simulink model "FarrowResamp"  (Simulink 6.6)
settings: Solver=VariableStepDiscrete  StartTime=0.0  StopTime=1800*clock_sample  RelTol=1e-3
PreLoadFcn:
  | clock_period=50/3
  | clock_sample=clock_period*1.0e-009
  | slow_clock=25
  | fast_clock=32
InitFcn:
  | %% DSPBuilder Start
  | alt_dspbuilder_update_model(bdroot)
  | %% DSPBuilder End
undefined symbols (not defined in the file): get
libraries: allblocks_alteradspbuilder2 x65, dspsnks4 x4
settings Model: Creator=mjervis  LastModifiedBy=lkong
settings DataIOCC: SignalLoggingName=sigsOut
settings OptimizationCC: InlineInvariantSignals=on
settings DebuggingCC: SignalResolutionControl=TryResolveAllWithWarning  SolverPrmCheckMsg=none  MultiTaskDSMMsg=warning  MultiTaskCondExecSysMsg=none  SigSpecEnsureSampleTimeMsg=none
settings HardwareCC: TargetUnknown=on
settings RTWCC: IncludeERTFirstTime=on

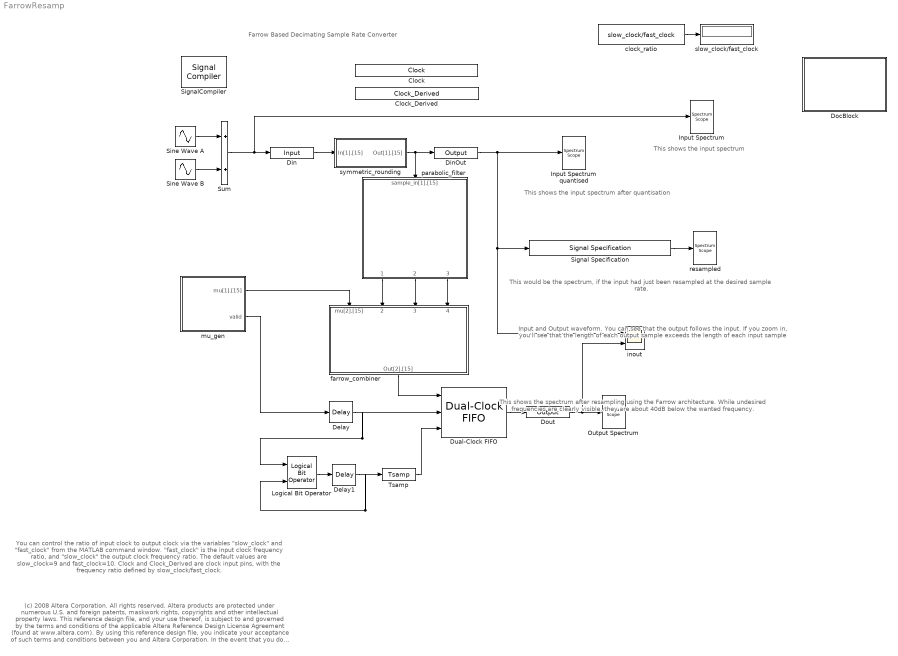
== system FarrowResamp ==
  note: (c) 2008 Altera Corporation. All rights reserved.  Altera products are protected under numerous U.S. and foreign patents, maskwork rights, copyrights and other intellectual property laws.
      | This reference design file, and your use thereof, is subject to and governed by the terms and conditions of the applicable Altera Reference Design License Agreement (found at www.altera.com).
      | By using this reference design file, you indicate your acceptance of such terms and conditions between you and Altera Corporation.
      | In the event that you do not agree with such terms and conditions, you may not use the reference design file and please promptly destroy any copies you have made.
      | This reference design file being provided on an "as-is" basis and as an accommodation and therefore all warranties, representations or guarantees of any kind (whether express, implied or statutory)
      | including, without limitation, warranties of merchantability, non-infringement, or fitness for a particular purpose, are specifically disclaimed.
      | By making this reference design file available, Altera expressly does not recommend, suggest or require that this reference design file be used in combination with any other product not provided by Altera
  note: This shows the input spectrum
  note: This shows the input spectrum after quantisation
  note: This shows the spectrum after resampling using the Farrow
      | architecture.  While undesired frequencies are clearly visible,
      | they are about 40dB below the wanted frequency.
  note: You can control the ratio of input clock to output clock via the variables "slow_clock" and "fast_clock" from the
      | MATLAB command window.  "fast_clock" is the input clock frequency ratio, and "slow_clock" the output clock
      | frequency ratio. The default values are slow_clock=9 and fast_clock=10.
      |
      | Clock and Clock_Derived are clock input pins, with the frequency ratio defined by slow_clock/fast_clock.
  note: Farrow Based Decimating Sample Rate Converter
  note: This would be the spectrum, if the input had
      | just been resampled at the desired sample rate.
  note: Input and Output waveform.  You can see that the output
      | follows the input.  If you zoom in, you'll see that the length
      | of each output sample exceeds the length of each input
      | sample
  Clock : allblocks_alteradspbuilder2/Clock  ClockPeriod=clock_period  ClockPeriodUnit=ns  SampleTime=clock_sample  SimulationStartCycle=5  PhaseOffset=0  Reset=aclr  ResetType=Active Low  Export=off
  Clock_Derived : allblocks_alteradspbuilder2/Clock_Derived  ClockNumerator=slow_clock  ClockDenominator=fast_clock  SimulationStartCycle=5  PhaseOffset=0  Reset=slow_aclr  ResetType=Active Low  Export=off
  Delay : allblocks_alteradspbuilder2/Delay  pipeline=4  pipeline_display=4  ClockPhase=1  use_ena=off  use_sclr=off  allowFloatingPointOverride=on  logOutputs=off  logFile=d:\spr\269066\tb_FarrowResamp\FarrowResamp_Delay.fixedpointlog  use_init=off  reset_value=1
  Delay1 : allblocks_alteradspbuilder2/Delay  pipeline=4  pipeline_display=4  ClockPhase=1  use_ena=off  use_sclr=off  allowFloatingPointOverride=on  logOutputs=off  logFile=d:\spr\269066\tb_FarrowResamp\FarrowResamp_Delay1.fixedpointlog  use_init=off  reset_value=1
  Din : allblocks_alteradspbuilder2/Input  iofile=d:\spr\269066\tb_FarrowResamp\FarrowResamp_Din.salt  BusType=Signed Fractional  bwl=1  bwr=15  SpecifyClock=on  clock=Clock  PORTTYPE=Input  externalType=Inferred  allowFloatingPointOverride=on  logOutputs=off
  DinOut : allblocks_alteradspbuilder2/Output  iofile=d:\spr\269066\tb_FarrowResamp\FarrowResamp_DinOut.capture  BusType=Signed Fractional  bwl=1  bwr=15  externalType=Inferred  PORTTYPE=Output  allowFloatingPointOverride=on  logOutputs=off
  DocBlock : Subsystem  mask(DocBlock){ECoderFlag=, DocumentType=Text}
      content=|
      | =============================================
      | Farrow Based Decimating Sample Rate Converter
      | =============================================
      |
      | Introduction
      | ------------
      | Many integrated systems, such as Software Defined Radios (SDR), require data
      | to be resampled.  This is typically the case where a unit can be configured to
      | comply with different communication standards, where the sample rates are different.
      | In some cases, where one clock rate is a simple integer multiply of another clock
      | rate, this can be done with interpolating and decimating FIR filters.  However, in
      | most cases the interpolation and decimation factors would be so high that this
      | approach is impractical.
      | Farrow resamplers offer an efficient way to resample a data stream at a different
      | sample rate.  The underlying principle is that the phase difference between the
      | current input and wanted output is determined on a sample by sample basis.  This
      | phase difference is then used to combine the phases of a polyphase filter in such
      | a way that a sample for the wanted output phase is generated.
      | This design demonstrates how a Farrow resampler is working.  You can simulate its
      | performance in MATLAB, change it as required for your application, generate a
      | VDHL version and synthesize it to Altera devices.
      | This demo is designed for an input clock rate identical to the system clock.  For
      | applications where the input rate is much lower than the system clock, time sharing
      | should be implemented to get a cost effective solution.
      |
      |
      | Usage
      | -----
      | You can run the design as it is, just press the run button to start the simulation.
      | You will get 4 waveforms, showing the spectrum at the following places:
      | 1) the input
      | 2) the input, quantised
      | 3) the input, if it had been just resampledby registering it in a flip flop running
      |    at the output clock rate (the simplest way of changing sample rate)
      | 4) at the output of the Farrow resampler.
      |
      | You can generate VHDL and synthesise the same way as any other DSPBuilder design
      | using the "SignalCompiler" block.
      |
      | You can change the stimuli by connecting the input to a different source.  If you
      | want to change the ratio of input clock to output clock, you can do this from the
      | MATLAB command prompt.  In this case, please set the variables "slow_clock" and
      | "fast_clock" to the required numbers, by default they are set to 9 and 10 to provide
      | a ratio of 9/10, i.e. the output rate is 90% of the input clock rate.  The
      | variables "fast_clock" and "slow_clock" are used in a number of instances
      | throughout the design.  The rules for setting these variables are:
      | 1) slow_clock, i.e. the output clock, must be slower than fast_clock for a deci-
      |    mating Farrow filter.
      | 2) slow_clock*fast_clock must be less than 2^14.  This is a restriction of this
      |    particular implementation.  You can work with ratios where this is not the
      |    case, but you then need to change the bit width in the accumulators in the
      |    mu_gen block.
      | 3) If slow_clock is less than half of fast_clock, the filter will work, but
      |    the results will be sub-optimal.  In this case it is better to double slow_clock,
      |    which should then still be less than fast_clock, and decimate at the output by
      |    rejecting every other sample.
      |
      |
      | Design details
      | --------------
      |
      | Input Stimuli
      |
      |   This testbench provides three stimuli:
      |   1) The sinewave generator is useful to analyse the effect of the resampling on
      |      the frequency spectrum.   You can change the frequency by double-clicking
      |      the "Sine Wave" block, and changing the "Samples per Period" parameter.
      |   2) The impulse generator generates a single impulse and is 0 for the rest of the
      |      simulation.  This is a useful tool for investigating the filter, which is part
      |      of the farrow resampler.
      |   3) The addition of two sinewaves.
      |
      | Symmetric rounding
      |
      |   Symmetric rounding ensures that no DC offset is introduced through the
      |   rounding operation.
      |
      | Parabolic filter
      |
      |   Low pass filter with passband=0.25 and stopband=0.75 .  You find more detailed
      |   documentation when you push into the filter by double-clicking it.
      |
      | mu Generator
      |
      |   This block calculates the phase difference between the current input sample
      |   and the desired output sample.  Double-click for more information.
      |
      | Farrow Combiner
      |
      |   The farrow combiner replaces the polyphase selector in traditional polyphase
      |   filters.  It will weigh the individual polyphases before adding them.  Double-
      |   click the Farrow_Combiner block for more information.
      |
      | FIFO
      |
      |   The farrow combiner works at the input clock rate.  This means it generates more
      |   samples than it should.  The task of the FIFO is to remove invalid samples, and
      |   also allows the transfer between the clock domains.  While the write side works
      |   at input clock rate, the read side works at output clock rate.
      mask prompts: ECoderFlag "E Coder Flag"; DocumentType "Document Type"
      mask help: Use this block to save long descriptive text with the model. Double-clicking the block will open an editor.
      settings: CopyFcn=docblock('breaklink',gcb);  DeleteFcn=docblock('close_document',gcb);  PreSaveFcn=docblock('save_document',gcb);  OpenFcn=docblock('edit_document',gcb);
      mask StyleString: edit,popup(Text|RTF|HTML)
      mask Display:
      | plot([.8 0 0 1 1 .8 .8 1],[1 1 0 0 .8 1 .8 .8]);
      | text(.5,.5,'DOC','horizontalalignment','center');
  Dout : allblocks_alteradspbuilder2/Output  iofile=d:\spr\269066\tb_FarrowResamp\FarrowResamp_Dout.capture  BusType=Signed Fractional  bwl=2  bwr=15  externalType=Inferred  PORTTYPE=Output  allowFloatingPointOverride=on  logOutputs=off
  Dual-Clock FIFO : allblocks_alteradspbuilder2/Dual-Clock FIFO  numwords=16  BusType=Signed Fractional  bwl=2  bwr=15  ram_type=AUTO  UseBaseWriteClock=on  UseBaseReadClock=off  read_clock=Clock_Derived  use_rdempty=off  use_rdfull=off  use_rdusedw=off  use_wrempty=off  use_wrfull=off  use_wrusedw=off  use_user_aclr=off  register_output=off  use_les_only=off  showahead_mode=off  synchronized=off  allowFloatingPointOverride=on  logOutputs=off  logFile=d:\spr\269066\tb_FarrowResamp\FarrowResamp_Dual-Clock+FIFO.fixedpointlog
  Input Spectrum : dspsnks4/Spectrum Scope  DialogController=dspdialog.SpectrumScope  DialogControllerArgs=DataTag1  SystemSampleTime=-1  ScopeProperties=on  Domain=Frequency  HorizSpan=1  UseBuffer=on  BufferSize=1024  Overlap=512  inpFftLenInherit=off  FFTlength=128  numAvg=2  DisplayProperties=off  AxisGrid=on  Memory=off  FrameNumber=on  AxisLegend=off  AxisZoom=off  OpenScopeAtSimStart=on  OpenScopeImmediately=off  FigPos=get(0,'defaultfigureposition')  AxisProperties=off  XUnits=Hertz  XRange=[0...Fs/2]  InheritXIncr=on  XIncr=1.0  XLabel=Samples  XLimit=Auto  YUnits=dB  XMax=1  XMin=0  YLabel=Magnitude, dB  LineProperties=off  wintypeSpecScope=Hann  RsSpecScope=50  betaSpecScope=5  winsampSpecScope=Periodic
      settings: YMin=-153.243329043552  YMax=22.477497462716
  Input Spectrum quantised : dspsnks4/Spectrum Scope  DialogController=dspdialog.SpectrumScope  DialogControllerArgs=DataTag2  SystemSampleTime=-1  ScopeProperties=on  Domain=Frequency  HorizSpan=1  UseBuffer=on  BufferSize=1024  Overlap=512  inpFftLenInherit=off  FFTlength=128  numAvg=2  DisplayProperties=off  AxisGrid=on  Memory=off  FrameNumber=on  AxisLegend=off  AxisZoom=off  OpenScopeAtSimStart=on  OpenScopeImmediately=off  FigPos=get(0,'defaultfigureposition')  AxisProperties=off  XUnits=Hertz  XRange=[0...Fs/2]  InheritXIncr=on  XIncr=1.0  XLabel=Samples  XLimit=Auto  YUnits=dB  XMax=1  XMin=0  YLabel=Magnitude, dB  LineProperties=off  LineColors=magenta  wintypeSpecScope=Hann  RsSpecScope=50  betaSpecScope=5  winsampSpecScope=Periodic
      settings: YMin=-152.110626534928  YMax=22.4774480317679
  Logical Bit Operator : allblocks_alteradspbuilder2/Logical Bit Operator  LogicalOperator=OR  user_inputs=2  pipeline_display=0
  Output Spectrum : dspsnks4/Spectrum Scope  DialogController=dspdialog.SpectrumScope  DialogControllerArgs=DataTag3  SystemSampleTime=-1  ScopeProperties=on  Domain=Frequency  HorizSpan=1  UseBuffer=on  BufferSize=1024  Overlap=512  inpFftLenInherit=off  FFTlength=128  numAvg=2  DisplayProperties=off  AxisGrid=on  Memory=off  FrameNumber=on  AxisLegend=off  AxisZoom=off  OpenScopeAtSimStart=on  OpenScopeImmediately=off  FigPos=get(0,'defaultfigureposition')  AxisProperties=off  XUnits=Hertz  XRange=[0...Fs/2]  InheritXIncr=on  XIncr=1.0  XLabel=Samples  XLimit=Auto  YUnits=dB  XMax=1  XMin=0  YLabel=Magnitude, dB  LineProperties=off  LineColors=blue  wintypeSpecScope=Hann  RsSpecScope=50  betaSpecScope=5  winsampSpecScope=Periodic
      settings: YMin=-107.092610263266  YMax=23.1676114232961
  Signal Specification : SignalSpecification  SampleTime=clock_sample * (slow_clock/fast_clock)
  SignalCompiler : allblocks_alteradspbuilder2/Signal Compiler  DeviceFamily=Stratix III  DeviceName=AUTO  EnableSignalTap=off  SignalTapDepth=128  UseBoardBlock=off  StpUseDefaultClock=on  StpClock=clock  ExportDir=.
  Sine Wave A : Sin  SineType=Sample based  Amplitude=0.4999  SampleTime=clock_sample
  Sine Wave B : Sin  SineType=Sample based  Amplitude=0.4999  Samples=11  SampleTime=clock_sample
  Sum : Sum  SaturateOnIntegerOverflow=on
  Tsamp : allblocks_alteradspbuilder2/Tsamp  SpecifyClock=on  clock=Clock_Derived
  clock_ratio : Constant  Value=slow_clock/fast_clock
  farrow_combiner : Subsystem  Orientation=down  AncestorBlock=ALTELINK/AltLab/HDL SubSystem
      mask Type: SubSystem AlteraBlockSet
  inout : Scope  NumInputPorts=2
      settings: YMin=-5~-5  YMax=5~5  SaveName=ScopeData2
  mu_gen : Subsystem  AncestorBlock=ALTELINK/AltLab/HDL SubSystem
      mask Type: SubSystem AlteraBlockSet
  parabolic_filter : Subsystem  Orientation=down  AncestorBlock=ALTELINK/AltLab/HDL SubSystem
      mask Type: SubSystem AlteraBlockSet
  resampled : dspsnks4/Spectrum Scope  DialogController=dspdialog.SpectrumScope  DialogControllerArgs=DataTag4  SystemSampleTime=-1  ScopeProperties=on  Domain=Frequency  HorizSpan=1  UseBuffer=on  BufferSize=1024  Overlap=512  inpFftLenInherit=off  FFTlength=128  numAvg=2  DisplayProperties=off  AxisGrid=on  Memory=off  FrameNumber=on  AxisLegend=off  AxisZoom=off  OpenScopeAtSimStart=on  OpenScopeImmediately=off  FigPos=get(0,'defaultfigureposition')  AxisProperties=off  XUnits=Hertz  XRange=[0...Fs/2]  InheritXIncr=on  XIncr=1.0  XLabel=Samples  XLimit=Auto  YUnits=dB  XMax=1  XMin=0  YLabel=Magnitude, dB  LineProperties=off  LineColors=magenta  wintypeSpecScope=Hann  RsSpecScope=50  betaSpecScope=5  winsampSpecScope=Periodic
      settings: YMin=-152.110626534928  YMax=22.4774480317679
  slow_clock/fast_clock : Display
  symmetric_rounding : Subsystem  AncestorBlock=ALTELINK/AltLab/HDL SubSystem
      mask Type: SubSystem AlteraBlockSet
  wires:
  parabolic_filter/1(phase0[3].[15]) -> farrow_combiner/2(phase0[3].[15])
  parabolic_filter/2(phase1[3].[15]) -> farrow_combiner/3(phase1[3].[15])
  parabolic_filter/3(phase2[3].[15]) -> farrow_combiner/4(phase2[2].[15])
  mu_gen/1(mu[1].[15]) -> farrow_combiner/1(mu[2].[15])
  mu_gen/2(valid) -> Delay/1
  Delay/1 -> Dual-Clock FIFO/2, Logical Bit Operator/1
  Dout/1 -> Output Spectrum/1, inout/2
  Din/1 -> symmetric_rounding/1(In[1].[15])
  clock_ratio/1 -> slow_clock/fast_clock/1
  Sine Wave A/1 -> Sum/1
  Sine Wave B/1 -> Sum/2
  Signal Specification/1 -> resampled/1
  symmetric_rounding/1(Out[1].[15]) -> parabolic_filter/1(sample_in[1].[15]), DinOut/1
  Sum/1 -> Din/1, Input Spectrum/1
  DinOut/1 -> Input Spectrum quantised/1, inout/1, Signal Specification/1
  Logical Bit Operator/1 -> Delay1/1
  Delay1/1 -> Logical Bit Operator/2, Tsamp/1
  Tsamp/1 -> Dual-Clock FIFO/3
  Dual-Clock FIFO/1 -> Dout/1
  farrow_combiner/1(Out[2].[15]) -> Dual-Clock FIFO/1

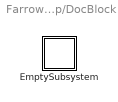
== system FarrowResamp/DocBlock ==
  EmptySubsystem : Subsystem

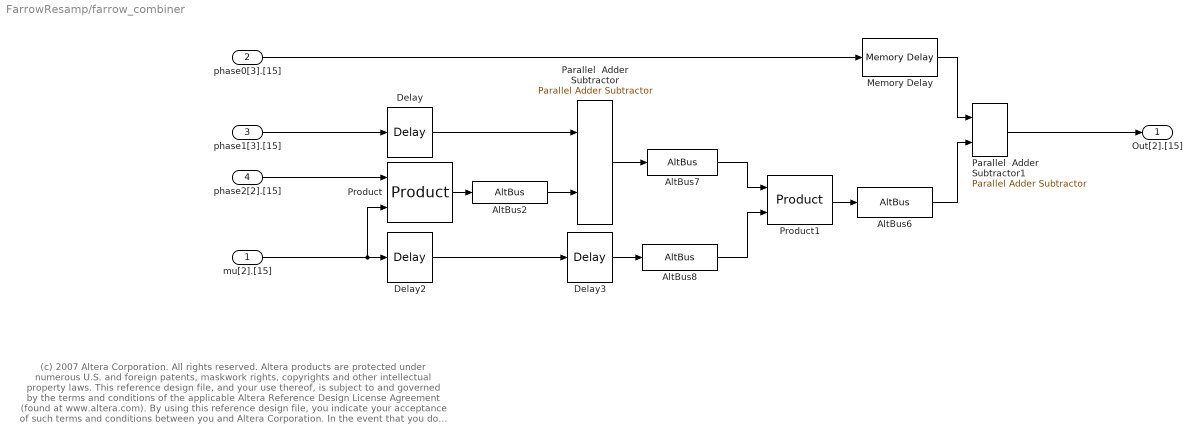
== system FarrowResamp/farrow_combiner ==
  note: (c) 2007 Altera Corporation. All rights reserved.  Altera products are protected under numerous U.S. and foreign patents, maskwork rights, copyrights and other intellectual property laws.
      | This reference design file, and your use thereof, is subject to and governed by the terms and conditions of the applicable Altera Reference Design License Agreement (found at www.altera.com).
      | By using this reference design file, you indicate your acceptance of such terms and conditions between you and Altera Corporation.
      | In the event that you do not agree with such terms and conditions, you may not use the reference design file and please promptly destroy any copies you have made.
      | This reference design file being provided on an "as-is" basis and as an accommodation and therefore all warranties, representations or guarantees of any kind (whether express, implied or statutory)
      | including, without limitation, warranties of merchantability, non-infringement, or fitness for a particular purpose, are specifically disclaimed.
      | By making this reference design file available, Altera expressly does not recommend, suggest or require that this reference design file be used in combination with any other product not provided by Altera
  mu[2].[15] : Inport
  phase0[3].[15] : Inport  Port=2
  phase1[3].[15] : Inport  Port=3
  phase2[2].[15] : Inport  Port=4
  AltBus2 : allblocks_alteradspbuilder2/AltBus  BusType=Signed Fractional  bwl=3  bwr=15  saturate=off  floatingPointInput=off  floatingPointOutput=off  logOutputs=off  logFile=d:\spr\269066\tb_FarrowResamp\FarrowResamp_farrow%5Fcombiner_AltBus2.fixedpointlog
  AltBus6 : allblocks_alteradspbuilder2/AltBus  BusType=Signed Fractional  bwl=5  bwr=15  saturate=off  floatingPointInput=off  floatingPointOutput=off  logOutputs=off  logFile=d:\spr\269066\tb_FarrowResamp\FarrowResamp_farrow%5Fcombiner_AltBus6.fixedpointlog
  AltBus7 : allblocks_alteradspbuilder2/AltBus  BusType=Signed Fractional  bwl=3  bwr=15  saturate=on  floatingPointInput=off  floatingPointOutput=off  logOutputs=off  logFile=d:\spr\269066\tb_FarrowResamp\FarrowResamp_farrow%5Fcombiner_AltBus7.fixedpointlog
  AltBus8 : allblocks_alteradspbuilder2/AltBus  BusType=Signed Fractional  bwl=2  bwr=15  saturate=off  floatingPointInput=off  floatingPointOutput=off  logOutputs=off  logFile=d:\spr\269066\tb_FarrowResamp\FarrowResamp_farrow%5Fcombiner_AltBus8.fixedpointlog
  Delay : allblocks_alteradspbuilder2/Delay  pipeline=1  pipeline_display=1  ClockPhase=1  use_ena=off  use_sclr=off  allowFloatingPointOverride=on  logOutputs=off  logFile=d:\spr\269066\tb_FarrowResamp\FarrowResamp_farrow%5Fcombiner_Delay.fixedpointlog  use_init=off  reset_value=1
  Delay2 : allblocks_alteradspbuilder2/Delay  pipeline=1  pipeline_display=1  ClockPhase=1  use_ena=off  use_sclr=off  allowFloatingPointOverride=on  logOutputs=off  logFile=d:\spr\269066\tb_FarrowResamp\FarrowResamp_farrow%5Fcombiner_Delay2.fixedpointlog  use_init=off  reset_value=1
  Delay3 : allblocks_alteradspbuilder2/Delay  pipeline=1  pipeline_display=1  ClockPhase=1  use_ena=off  use_sclr=off  allowFloatingPointOverride=on  logOutputs=off  logFile=d:\spr\269066\tb_FarrowResamp\FarrowResamp_farrow%5Fcombiner_Delay3.fixedpointlog  use_init=off  reset_value=1
  Memory Delay : allblocks_alteradspbuilder2/Memory Delay  BusType=Inferred  bwl=8  bwr=0  pipeline=3  pipeline_display=3  ram_type=AUTO  use_ena=off  use_sclr=off  allowFloatingPointOverride=on  logOutputs=off  logFile=d:\spr\269066\tb_FarrowResamp\FarrowResamp_farrow%5Fcombiner_Memory+Delay.fixedpointlog
  Parallel  Adder Subtractor : allblocks_alteradspbuilder2/Parallel Adder Subtractor  number_of_inputs=2  direction=++  use_pipeline=on  pipeline_display=1  phase_selection=1  use_ena=off  use_aclr=off  allowFloatingPointOverride=on  logOutputs=off  logFile=d:\spr\269066\tb_FarrowResamp\FarrowResamp_farrow%5Fcombiner_Parallel+%0AAdder+Subtractor.fixedpointlog
  Parallel  Adder Subtractor1 : allblocks_alteradspbuilder2/Parallel Adder Subtractor  number_of_inputs=2  direction=++  use_pipeline=on  pipeline_display=1  phase_selection=1  use_ena=off  use_aclr=off  allowFloatingPointOverride=on  logOutputs=off  logFile=d:\spr\269066\tb_FarrowResamp\FarrowResamp_farrow%5Fcombiner_Parallel+%0AAdder+Subtractor1.fixedpointlog
  Product : allblocks_alteradspbuilder2/Product  BusType=Inferred  bwl=8  bwr=0  pipeline=1  pipeline_display=1  phase_selection=1  use_ena=off  use_aclr=off  UseLPM=off  UseDedicatedCircuitry=off  allowFloatingPointOverride=on  logOutputs=off  logFile=d:\spr\269066\tb_FarrowResamp\FarrowResamp_farrow%5Fcombiner_Product.fixedpointlog
  Product1 : allblocks_alteradspbuilder2/Product  BusType=Inferred  bwl=8  bwr=0  pipeline=1  pipeline_display=1  phase_selection=1  use_ena=off  use_aclr=off  UseLPM=off  UseDedicatedCircuitry=off  allowFloatingPointOverride=on  logOutputs=off  logFile=d:\spr\269066\tb_FarrowResamp\FarrowResamp_farrow%5Fcombiner_Product1.fixedpointlog
  Out[2].[15] : Outport
  wires:
  phase0[3].[15]/1 -> Memory Delay/1
  phase1[3].[15]/1 -> Delay/1
  phase2[2].[15]/1 -> Product/1
  mu[2].[15]/1 -> Product/2, Delay2/1
  Delay/1 -> Parallel  Adder Subtractor/1
  Product/1 -> AltBus2/1
  Parallel  Adder Subtractor/1 -> AltBus7/1
  Delay2/1 -> Delay3/1
  Product1/1 -> AltBus6/1
  Delay3/1 -> AltBus8/1
  AltBus8/1 -> Product1/2
  AltBus6/1 -> Parallel  Adder Subtractor1/2
  AltBus7/1 -> Product1/1
  Parallel  Adder Subtractor1/1 -> Out[2].[15]/1
  Memory Delay/1 -> Parallel  Adder Subtractor1/1
  AltBus2/1 -> Parallel  Adder Subtractor/2

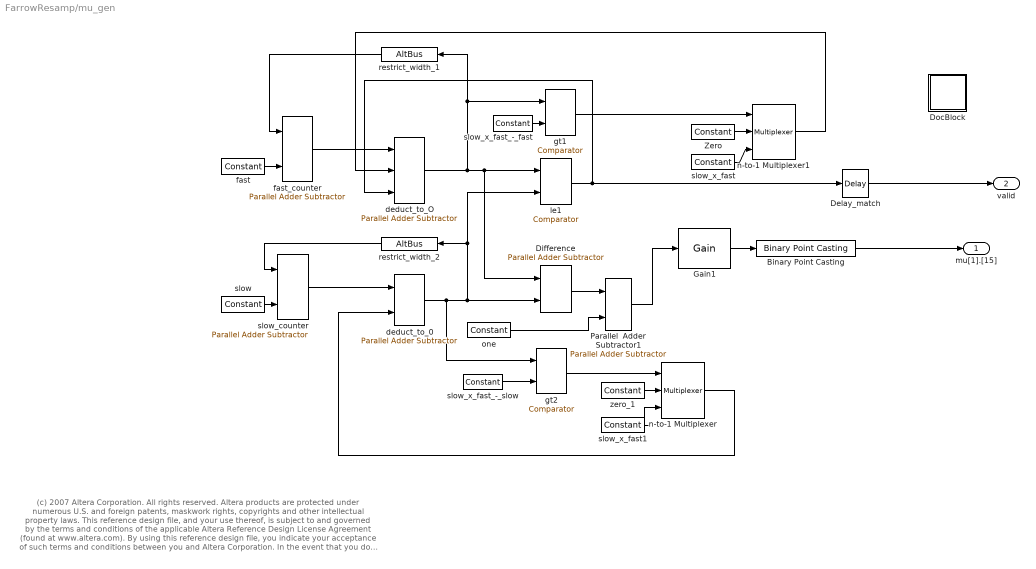
== system FarrowResamp/mu_gen ==
  note: (c) 2007 Altera Corporation. All rights reserved.  Altera products are protected under numerous U.S. and foreign patents, maskwork rights, copyrights and other intellectual property laws.
      | This reference design file, and your use thereof, is subject to and governed by the terms and conditions of the applicable Altera Reference Design License Agreement (found at www.altera.com).
      | By using this reference design file, you indicate your acceptance of such terms and conditions between you and Altera Corporation.
      | In the event that you do not agree with such terms and conditions, you may not use the reference design file and please promptly destroy any copies you have made.
      | This reference design file being provided on an "as-is" basis and as an accommodation and therefore all warranties, representations or guarantees of any kind (whether express, implied or statutory)
      | including, without limitation, warranties of merchantability, non-infringement, or fitness for a particular purpose, are specifically disclaimed.
      | By making this reference design file available, Altera expressly does not recommend, suggest or require that this reference design file be used in combination with any other product not provided by Altera
  Binary Point Casting : allblocks_alteradspbuilder2/Binary Point Casting  BusType=Signed Fractional  bwl=32  bwr=0  OutputPointPosition=15  pipeline_display=0
  Delay_match : allblocks_alteradspbuilder2/Delay  pipeline=3  pipeline_display=3  ClockPhase=1  use_ena=off  use_sclr=off  allowFloatingPointOverride=on  logOutputs=off  logFile=d:\spr\269066\tb_FarrowResamp\FarrowResamp_mu%5Fgen_Delay%5Fmatch.fixedpointlog  use_init=off  reset_value=1
  Difference : allblocks_alteradspbuilder2/Parallel Adder Subtractor  number_of_inputs=2  direction=-  use_pipeline=on  pipeline_display=1  phase_selection=1  use_ena=off  use_aclr=off  allowFloatingPointOverride=on  logOutputs=off  logFile=d:\spr\269066\tb_FarrowResamp\FarrowResamp_mu%5Fgen_Difference.fixedpointlog
  DocBlock : Subsystem  mask(DocBlock){ECoderFlag=, DocumentType=Text}
      mask prompts: ECoderFlag "E Coder Flag"; DocumentType "Document Type"
      mask help: Use this block to save long descriptive text with the model. Double-clicking the block will open an editor.
      settings: CopyFcn=docblock('breaklink',gcb);  DeleteFcn=docblock('close_document',gcb);  PreSaveFcn=docblock('save_document',gcb);  OpenFcn=docblock('edit_document',gcb);
      mask StyleString: edit,popup(Text|RTF|HTML)
      mask Display:
      | plot([.8 0 0 1 1 .8 .8 1],[1 1 0 0 .8 1 .8 .8]);
      | text(.5,.5,'DOC','horizontalalignment','center');
  Gain1 : allblocks_alteradspbuilder2/Gain  vgain=(1/slow_clock+2^-15) *(2^15)  BusType=Signed Integer  bwl=16  bwr=0  pipeline=2  pipeline_display=2  allowFloatingPointOverride=on  logOutputs=off  logFile=d:\spr\269066\tb_FarrowResamp\FarrowResamp_mu%5Fgen_Gain1.fixedpointlog  use_ena=off  use_aclr=off  lpm=off  MaskValue=1
  Parallel  Adder Subtractor1 : allblocks_alteradspbuilder2/Parallel Adder Subtractor  number_of_inputs=2  direction=++  use_pipeline=off  pipeline_display=0  phase_selection=1  use_ena=on  use_aclr=on  allowFloatingPointOverride=on  logOutputs=off  logFile=d:\spr\269066\tb_FarrowResamp\FarrowResamp_mu%5Fgen_Parallel+%0AAdder+Subtractor1.fixedpointlog
  Zero : allblocks_alteradspbuilder2/Constant  mask_cst=0  BusType=Signed Integer  bwl=12  bwr=0  roundMode=Truncate  satMode=Wrap  SpecifyClock=off  allowFloatingPointOverride=on  logOutputs=off  logFile=d:\spr\269066\tb_FarrowResamp\FarrowResamp_mu%5Fgen_Zero.fixedpointlog
  deduct_to_0 : allblocks_alteradspbuilder2/Parallel Adder Subtractor  number_of_inputs=2  direction=+-  use_pipeline=on  pipeline_display=1  phase_selection=1  use_ena=off  use_aclr=off  allowFloatingPointOverride=on  logOutputs=off  logFile=d:\spr\269066\tb_FarrowResamp\FarrowResamp_mu%5Fgen_deduct%5Fto%5F0.fixedpointlog
  deduct_to_O : allblocks_alteradspbuilder2/Parallel Adder Subtractor  number_of_inputs=2  direction=+-  use_pipeline=on  pipeline_display=1  phase_selection=1  use_ena=on  use_aclr=off  allowFloatingPointOverride=on  logOutputs=off  logFile=d:\spr\269066\tb_FarrowResamp\FarrowResamp_mu%5Fgen_deduct%5Fto%5FO.fixedpointlog
  fast : allblocks_alteradspbuilder2/Constant  mask_cst=fast_clock  BusType=Signed Integer  bwl=12  bwr=0  roundMode=Truncate  satMode=Wrap  SpecifyClock=off  allowFloatingPointOverride=on  logOutputs=off  logFile=d:\spr\269066\tb_FarrowResamp\FarrowResamp_mu%5Fgen_fast.fixedpointlog
  fast_counter : allblocks_alteradspbuilder2/Parallel Adder Subtractor  number_of_inputs=2  direction=+  use_pipeline=off  pipeline_display=0  phase_selection=1  use_ena=on  use_aclr=on  allowFloatingPointOverride=on  logOutputs=off  logFile=d:\spr\269066\tb_FarrowResamp\FarrowResamp_mu%5Fgen_fast%5Fcounter.fixedpointlog
  gt1 : allblocks_alteradspbuilder2/Comparator  direction=a > b  pipeline_display=0  allowFloatingPointOverride=on  logOutputs=off  logFile=d:\spr\269066\tb_FarrowResamp\FarrowResamp_mu%5Fgen_gt1.fixedpointlog
  gt2 : allblocks_alteradspbuilder2/Comparator  direction=a > b  pipeline_display=0  allowFloatingPointOverride=on  logOutputs=off  logFile=d:\spr\269066\tb_FarrowResamp\FarrowResamp_mu%5Fgen_gt2.fixedpointlog
  le1 : allblocks_alteradspbuilder2/Comparator  direction=a <= b  pipeline_display=0  allowFloatingPointOverride=on  logOutputs=off  logFile=d:\spr\269066\tb_FarrowResamp\FarrowResamp_mu%5Fgen_le1.fixedpointlog
  n-to-1 Multiplexer : allblocks_alteradspbuilder2/Multiplexer  numInputs=2  pipeline=0  oneHot=off  pipeline_display=0  use_ena=off  use_aclr=off  allowFloatingPointOverride=on  logOutputs=off  logFile=d:\spr\269066\tb_FarrowResamp\FarrowResamp_mu%5Fgen_n-to-1+Multiplexer.fixedpointlog
  n-to-1 Multiplexer1 : allblocks_alteradspbuilder2/Multiplexer  numInputs=2  pipeline=0  oneHot=off  pipeline_display=0  use_ena=off  use_aclr=off  allowFloatingPointOverride=on  logOutputs=off  logFile=d:\spr\269066\tb_FarrowResamp\FarrowResamp_mu%5Fgen_n-to-1+Multiplexer1.fixedpointlog
  one : allblocks_alteradspbuilder2/Constant  mask_cst=1  BusType=Signed Integer  bwl=12  bwr=0  roundMode=Truncate  satMode=Wrap  SpecifyClock=off  allowFloatingPointOverride=on  logOutputs=off  logFile=d:\spr\269066\tb_FarrowResamp\FarrowResamp_mu%5Fgen_one.fixedpointlog
  restrict_width_1 : allblocks_alteradspbuilder2/AltBus  Orientation=left  BusType=Signed Integer  bwl=14  bwr=0  saturate=off  floatingPointInput=off  floatingPointOutput=off  logOutputs=off  logFile=d:\spr\269066\tb_FarrowResamp\FarrowResamp_mu%5Fgen_restrict%5Fwidth%5F1.fixedpointlog
  restrict_width_2 : allblocks_alteradspbuilder2/AltBus  Orientation=left  BusType=Signed Integer  bwl=14  bwr=0  saturate=off  floatingPointInput=off  floatingPointOutput=off  logOutputs=off  logFile=d:\spr\269066\tb_FarrowResamp\FarrowResamp_mu%5Fgen_restrict%5Fwidth%5F2.fixedpointlog
  slow : allblocks_alteradspbuilder2/Constant  mask_cst=slow_clock  BusType=Signed Integer  bwl=12  bwr=0  roundMode=Truncate  satMode=Wrap  SpecifyClock=off  allowFloatingPointOverride=on  logOutputs=off  logFile=d:\spr\269066\tb_FarrowResamp\FarrowResamp_mu%5Fgen_slow.fixedpointlog
  slow_counter : allblocks_alteradspbuilder2/Parallel Adder Subtractor  number_of_inputs=2  direction=+  use_pipeline=off  pipeline_display=0  phase_selection=1  use_ena=on  use_aclr=on  allowFloatingPointOverride=on  logOutputs=off  logFile=d:\spr\269066\tb_FarrowResamp\FarrowResamp_mu%5Fgen_slow%5Fcounter.fixedpointlog
  slow_x_fast : allblocks_alteradspbuilder2/Constant  mask_cst=slow_clock*fast_clock  BusType=Signed Integer  bwl=12  bwr=0  roundMode=Truncate  satMode=Wrap  SpecifyClock=off  allowFloatingPointOverride=on  logOutputs=off  logFile=d:\spr\269066\tb_FarrowResamp\FarrowResamp_mu%5Fgen_slow%5Fx%5Ffast.fixedpointlog
  slow_x_fast1 : allblocks_alteradspbuilder2/Constant  mask_cst=slow_clock*fast_clock  BusType=Signed Integer  bwl=12  bwr=0  roundMode=Truncate  satMode=Wrap  SpecifyClock=off  allowFloatingPointOverride=on  logOutputs=off  logFile=d:\spr\269066\tb_FarrowResamp\FarrowResamp_mu%5Fgen_slow%5Fx%5Ffast1.fixedpointlog
  slow_x_fast_-_fast : allblocks_alteradspbuilder2/Constant  mask_cst=slow_clock*fast_clock-fast_clock  BusType=Signed Integer  bwl=12  bwr=0  roundMode=Truncate  satMode=Wrap  SpecifyClock=off  allowFloatingPointOverride=on  logOutputs=off  logFile=d:\spr\269066\tb_FarrowResamp\FarrowResamp_mu%5Fgen_slow%5Fx%5Ffast%5F-%5Ffast.fixedpointlog
  slow_x_fast_-_slow : allblocks_alteradspbuilder2/Constant  mask_cst=slow_clock*fast_clock-slow_clock  BusType=Signed Integer  bwl=12  bwr=0  roundMode=Truncate  satMode=Wrap  SpecifyClock=off  allowFloatingPointOverride=on  logOutputs=off  logFile=d:\spr\269066\tb_FarrowResamp\FarrowResamp_mu%5Fgen_slow%5Fx%5Ffast%5F-%5Fslow.fixedpointlog
  zero_1 : allblocks_alteradspbuilder2/Constant  mask_cst=0  BusType=Signed Integer  bwl=12  bwr=0  roundMode=Truncate  satMode=Wrap  SpecifyClock=off  allowFloatingPointOverride=on  logOutputs=off  logFile=d:\spr\269066\tb_FarrowResamp\FarrowResamp_mu%5Fgen_zero%5F1.fixedpointlog
  mu[1].[15] : Outport
  valid : Outport  Port=2
  wires:
  deduct_to_0/1 -> restrict_width_2/1, le1/2, Difference/2, gt2/1
  deduct_to_O/1 -> restrict_width_1/1, gt1/1, le1/1, Difference/1
  le1/1 -> deduct_to_O/3, Delay_match/1
  gt2/1 -> n-to-1 Multiplexer/1
  zero_1/1 -> n-to-1 Multiplexer/2
  n-to-1 Multiplexer/1 -> deduct_to_0/2
  Zero/1 -> n-to-1 Multiplexer1/2
  gt1/1 -> n-to-1 Multiplexer1/1
  slow_x_fast1/1 -> n-to-1 Multiplexer/3
  slow_x_fast/1 -> n-to-1 Multiplexer1/3
  slow_x_fast_-_slow/1 -> gt2/2
  slow_x_fast_-_fast/1 -> gt1/2
  Delay_match/1 -> valid/1
  restrict_width_2/1 -> slow_counter/1
  slow/1 -> slow_counter/2
  slow_counter/1 -> deduct_to_0/1
  n-to-1 Multiplexer1/1 -> deduct_to_O/2
  fast_counter/1 -> deduct_to_O/1
  restrict_width_1/1 -> fast_counter/1
  fast/1 -> fast_counter/2
  Difference/1 -> Parallel  Adder Subtractor1/1
  Parallel  Adder Subtractor1/1 -> Gain1/1
  one/1 -> Parallel  Adder Subtractor1/2
  Gain1/1 -> Binary Point Casting/1
  Binary Point Casting/1 -> mu[1].[15]/1

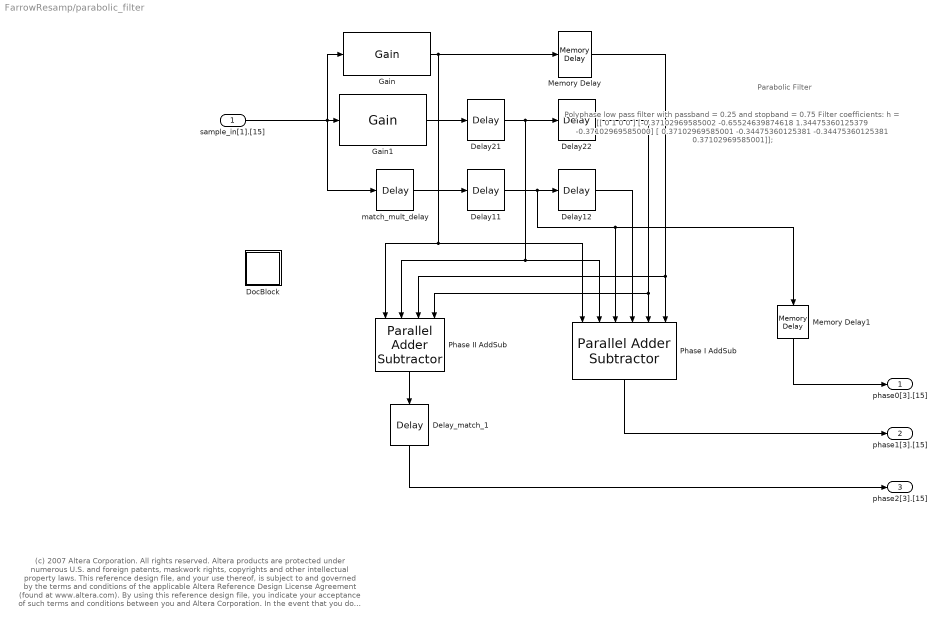
== system FarrowResamp/parabolic_filter ==
  note: Parabolic Filter
  note: Polyphase low pass filter with passband = 0.25 and stopband = 0.75
      |
      | Filter coefficients:
      | h = [[ 0                              1                                0                               0           ]
      |        [-0.37102969585002 -0.65524639874618  1.34475360125379 -0.37102969585000]
      |        [ 0.37102969585001 -0.34475360125381 -0.34475360125381  0.37102969585001]];
  note: (c) 2007 Altera Corporation. All rights reserved.  Altera products are protected under numerous U.S. and foreign patents, maskwork rights, copyrights and other intellectual property laws.
      | This reference design file, and your use thereof, is subject to and governed by the terms and conditions of the applicable Altera Reference Design License Agreement (found at www.altera.com).
      | By using this reference design file, you indicate your acceptance of such terms and conditions between you and Altera Corporation.
      | In the event that you do not agree with such terms and conditions, you may not use the reference design file and please promptly destroy any copies you have made.
      | This reference design file being provided on an "as-is" basis and as an accommodation and therefore all warranties, representations or guarantees of any kind (whether express, implied or statutory)
      | including, without limitation, warranties of merchantability, non-infringement, or fitness for a particular purpose, are specifically disclaimed.
      | By making this reference design file available, Altera expressly does not recommend, suggest or require that this reference design file be used in combination with any other product not provided by Altera
  sample_in[1].[15] : Inport
  Delay11 : allblocks_alteradspbuilder2/Delay  pipeline=1  pipeline_display=1  ClockPhase=1  use_ena=off  use_sclr=off  allowFloatingPointOverride=on  logOutputs=off  logFile=d:\spr\269066\tb_FarrowResamp\FarrowResamp_parabolic%5Ffilter_Delay11.fixedpointlog  use_init=off  reset_value=1
  Delay12 : allblocks_alteradspbuilder2/Delay  pipeline=1  pipeline_display=1  ClockPhase=1  use_ena=off  use_sclr=off  allowFloatingPointOverride=on  logOutputs=off  logFile=d:\spr\269066\tb_FarrowResamp\FarrowResamp_parabolic%5Ffilter_Delay12.fixedpointlog  use_init=off  reset_value=1
  Delay21 : allblocks_alteradspbuilder2/Delay  pipeline=1  pipeline_display=1  ClockPhase=1  use_ena=off  use_sclr=off  allowFloatingPointOverride=on  logOutputs=off  logFile=d:\spr\269066\tb_FarrowResamp\FarrowResamp_parabolic%5Ffilter_Delay21.fixedpointlog  use_init=off  reset_value=1
  Delay22 : allblocks_alteradspbuilder2/Delay  pipeline=1  pipeline_display=1  ClockPhase=1  use_ena=off  use_sclr=off  allowFloatingPointOverride=on  logOutputs=off  logFile=d:\spr\269066\tb_FarrowResamp\FarrowResamp_parabolic%5Ffilter_Delay22.fixedpointlog  use_init=off  reset_value=1
  Delay_match_1 : allblocks_alteradspbuilder2/Delay  Orientation=down  pipeline=1  pipeline_display=1  ClockPhase=1  use_ena=off  use_sclr=off  allowFloatingPointOverride=on  logOutputs=off  logFile=d:\spr\269066\tb_FarrowResamp\FarrowResamp_parabolic%5Ffilter_Delay%5Fmatch%5F1.fixedpointlog  use_init=off  reset_value=1
  DocBlock : Subsystem  mask(DocBlock){ECoderFlag=, DocumentType=Text}
      mask prompts: ECoderFlag "E Coder Flag"; DocumentType "Document Type"
      mask help: Use this block to save long descriptive text with the model. Double-clicking the block will open an editor.
      settings: CopyFcn=docblock('breaklink',gcb);  DeleteFcn=docblock('close_document',gcb);  PreSaveFcn=docblock('save_document',gcb);  OpenFcn=docblock('edit_document',gcb);
      mask StyleString: edit,popup(Text|RTF|HTML)
      mask Display:
      | plot([.8 0 0 1 1 .8 .8 1],[1 1 0 0 .8 1 .8 .8]);
      | text(.5,.5,'DOC','horizontalalignment','center');
  Gain : allblocks_alteradspbuilder2/Gain  vgain=0.37102969585002  BusType=Signed Fractional  bwl=1  bwr=15  pipeline=1  pipeline_display=1  allowFloatingPointOverride=on  logOutputs=off  logFile=d:\spr\269066\tb_FarrowResamp\FarrowResamp_parabolic%5Ffilter_Gain.fixedpointlog  use_ena=off  use_aclr=off  lpm=off  MaskValue=1
  Gain1 : allblocks_alteradspbuilder2/Gain  vgain=0.34475360125381  BusType=Signed Fractional  bwl=1  bwr=15  pipeline=1  pipeline_display=1  allowFloatingPointOverride=on  logOutputs=off  logFile=d:\spr\269066\tb_FarrowResamp\FarrowResamp_parabolic%5Ffilter_Gain1.fixedpointlog  use_ena=off  use_aclr=off  lpm=off  MaskValue=1
  Memory Delay : allblocks_alteradspbuilder2/Memory Delay  BusType=Inferred  bwl=8  bwr=0  pipeline=3  pipeline_display=3  ram_type=AUTO  use_ena=off  use_sclr=off  allowFloatingPointOverride=on  logOutputs=off  logFile=d:\spr\269066\tb_FarrowResamp\FarrowResamp_parabolic%5Ffilter_Memory+Delay.fixedpointlog
  Memory Delay1 : allblocks_alteradspbuilder2/Memory Delay  Orientation=down  BusType=Inferred  bwl=8  bwr=0  pipeline=3  pipeline_display=3  ram_type=AUTO  use_ena=off  use_sclr=off  allowFloatingPointOverride=on  logOutputs=off  logFile=d:\spr\269066\tb_FarrowResamp\FarrowResamp_parabolic%5Ffilter_Memory+Delay1.fixedpointlog
  Phase I AddSub : allblocks_alteradspbuilder2/Parallel Adder Subtractor  Orientation=down  number_of_inputs=6  direction=-+-++-  use_pipeline=on  pipeline_display=3  phase_selection=1  use_ena=off  use_aclr=off  allowFloatingPointOverride=on  logOutputs=off  logFile=d:\spr\269066\tb_FarrowResamp\FarrowResamp_parabolic%5Ffilter_Phase+I+AddSub.fixedpointlog
  Phase II AddSub : allblocks_alteradspbuilder2/Parallel Adder Subtractor  Orientation=down  number_of_inputs=4  direction=+-+-  use_pipeline=on  pipeline_display=2  phase_selection=1  use_ena=off  use_aclr=off  allowFloatingPointOverride=on  logOutputs=off  logFile=d:\spr\269066\tb_FarrowResamp\FarrowResamp_parabolic%5Ffilter_Phase+II+AddSub.fixedpointlog
  match_mult_delay : allblocks_alteradspbuilder2/Delay  pipeline=1  pipeline_display=1  ClockPhase=1  use_ena=off  use_sclr=off  allowFloatingPointOverride=on  logOutputs=off  logFile=d:\spr\269066\tb_FarrowResamp\FarrowResamp_parabolic%5Ffilter_match%5Fmult%5Fdelay.fixedpointlog  use_init=off  reset_value=1
  phase0[3].[15] : Outport
  phase1[3].[15] : Outport  Port=2
  phase2[3].[15] : Outport  Port=3
  wires:
  sample_in[1].[15]/1 -> Gain/1, match_mult_delay/1, Gain1/1
  Delay21/1 -> Delay22/1, Phase II AddSub/2, Phase I AddSub/2
  Delay22/1 -> Phase II AddSub/4, Phase I AddSub/5
  Delay11/1 -> Delay12/1, Phase I AddSub/3, Memory Delay1/1
  Gain/1 -> Phase II AddSub/1, Phase I AddSub/1, Memory Delay/1
  Gain1/1 -> Delay21/1
  match_mult_delay/1 -> Delay11/1
  Memory Delay/1 -> Phase II AddSub/3, Phase I AddSub/6
  Memory Delay1/1 -> phase0[3].[15]/1
  Phase I AddSub/1 -> phase1[3].[15]/1
  Phase II AddSub/1 -> Delay_match_1/1
  Delay_match_1/1 -> phase2[3].[15]/1
  Delay12/1 -> Phase I AddSub/4

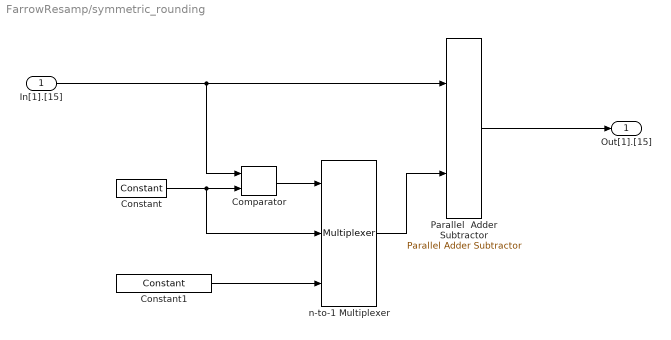
== system FarrowResamp/symmetric_rounding ==
  In[1].[15] : Inport
  Comparator : allblocks_alteradspbuilder2/Comparator  direction=a < b  pipeline_display=0  allowFloatingPointOverride=on  logOutputs=off  logFile=d:\spr\269066\tb_FarrowResamp\FarrowResamp_symmetric%5Frounding_Comparator.fixedpointlog
  Constant : allblocks_alteradspbuilder2/Constant  mask_cst=0  BusType=Signed Fractional  bwl=1  bwr=15  roundMode=Truncate  satMode=Wrap  SpecifyClock=off  allowFloatingPointOverride=on  logOutputs=off  logFile=d:\spr\269066\tb_FarrowResamp\FarrowResamp_symmetric%5Frounding_Constant.fixedpointlog
  Constant1 : allblocks_alteradspbuilder2/Constant  mask_cst=1*2^-15  BusType=Signed Fractional  bwl=1  bwr=15  roundMode=Truncate  satMode=Wrap  SpecifyClock=off  allowFloatingPointOverride=on  logOutputs=off  logFile=d:\spr\269066\tb_FarrowResamp\FarrowResamp_symmetric%5Frounding_Constant1.fixedpointlog
  Parallel  Adder Subtractor : allblocks_alteradspbuilder2/Parallel Adder Subtractor  number_of_inputs=2  direction=+  use_pipeline=on  pipeline_display=1  phase_selection=1  use_ena=off  use_aclr=off  allowFloatingPointOverride=on  logOutputs=off  logFile=d:\spr\269066\tb_FarrowResamp\FarrowResamp_symmetric%5Frounding_Parallel+%0AAdder+Subtractor.fixedpointlog
  n-to-1 Multiplexer : allblocks_alteradspbuilder2/Multiplexer  numInputs=2  pipeline=0  oneHot=off  pipeline_display=0  use_ena=off  use_aclr=off  allowFloatingPointOverride=on  logOutputs=off  logFile=d:\spr\269066\tb_FarrowResamp\FarrowResamp_symmetric%5Frounding_n-to-1+Multiplexer.fixedpointlog
  Out[1].[15] : Outport
  wires:
  In[1].[15]/1 -> Comparator/1, Parallel  Adder Subtractor/1
  Constant/1 -> n-to-1 Multiplexer/2, Comparator/2
  Comparator/1 -> n-to-1 Multiplexer/1
  Constant1/1 -> n-to-1 Multiplexer/3
  Parallel  Adder Subtractor/1 -> Out[1].[15]/1
  n-to-1 Multiplexer/1 -> Parallel  Adder Subtractor/2

== system FarrowResamp/DocBlock/EmptySubsystem ==

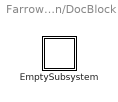
== system FarrowResamp/mu_gen/DocBlock ==
  EmptySubsystem : Subsystem

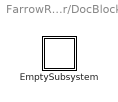
== system FarrowResamp/parabolic_filter/DocBlock ==
  EmptySubsystem : Subsystem

== system FarrowResamp/mu_gen/DocBlock/EmptySubsystem ==

== system FarrowResamp/parabolic_filter/DocBlock/EmptySubsystem ==
